simulink model "retard"  (R2018b)
settings: Solver=VariableStepAuto  StartTime=0.0  StopTime=10.0  RelTol=1e-3
settings Model: Creator=xpess  LastModifiedBy=xpess

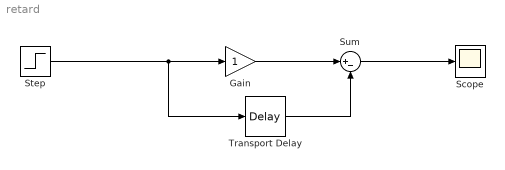
== system retard ==
  Gain : Gain
  Scope : Scope
  Step : Step  SampleTime=0
  Sum : Sum  Inputs=|+-
  Transport Delay : TransportDelay
  wires:
  Step/1 -> Transport Delay/1, Gain/1
  Gain/1 -> Sum/1
  Transport Delay/1 -> Sum/2
  Sum/1 -> Scope/1
